simulink model "torque_reflex"  (R2019b)
settings: Solver=ode4  StartTime=0.0  StopTime=inf  FixedStep=BKIN_STEP_TIME  RelTol=1e-3  EnableMultiTasking=on
StartFcn:
  |  warndlg('Dexterit-E models cannot run under simulation. Please compile your model and run it from within Dexterit-E.');set_param(bdroot,'SimulationCommand','stop')
model workspace (MAT data in the model file):
  ACTIVE = 4
  AMPLITUDE = 7
  BASE_STIFFNESS = 12
  BKIN_KINEMATIC_FRAME_SIZE = 400
  BKIN_STEP_TIME = 0.00025
  COLOR_2 = 5
  CONDITION = 3
  DELAY_POST_TRIAL = 4
  DURATION = 5
  E_END_TRIAL = 2
  E_HAND_OUT = 4
  E_NO_EVENT = 0
  E_SHOW_TARGET = 3
  E_SRS_ON = 6
  E_START_TRIAL = 5
  E_TARGET_REACHED = 1
  HAND_OUT_TIME = 6
  IMAGE = 3
  INSERT_OFFSET = 8
  L1_LENGTH = 6
  L1_LINE = 7
  L2_LENGTH = 7
  L2_LINE = 8
  LOAD = 2
  MOVE_THRESHOLD = 10
  MUSCLE = 1
  MUSCLE_LENGTH = 1
  REFLEX = 9
  REFLEX_GAIN = 5
  RESTING_FORCE = 2
  SPEED = 6
  SPRING_X = 1
  SPRING_Y = 2
  SRS_GAIN = 13
  TARGET_1 = 3
  THICKNESS = 4
  V_MAX = 3
  WALL_DAMPING = 11
  WALL_STIFFNESS = 9
  activation = 1
  col_x = 1
  col_y = 2
undefined symbols (not defined in the file or in its folder): slselsubs
libraries: Video x5, simulink x5, xpcutilitieslib x4, KINARM_IO x4, General x3, KINARM_loads x2, KINARM_EP_loads x2, KINARM_general x1, dspstat3 x1
(part 2 of 2)

== matlab function torque_reflex/Limb Mechanics /Integrate Signals ==
  settings: fimath=|
      | fimath(...
      | 'RoundMode', 'floor',...
      | 'OverflowMode', 'wrap',...
      | 'ProductMode', 'KeepLSB', 'ProductWordLength', 32,...
      | 'SumMode', 'KeepLSB', 'SumWordLength', 32,...
      | 'CastBeforeSum', false)
  data: t_0 input; rest_length input; Force input; hand_forces output; L2_offset input; force_SRS input; d input; L2 input; spring_constant input; FS input; muscle_vector input; out_angle output; force_muscle output
function [hand_forces, out_angle, force_muscle] = hill_forces(t_0, rest_length, Force, L2_offset, force_SRS, d, L2, spring_constant, FS, muscle_vector)
% spring_force = spring_constant * (rest_length - spring_length);
% spring_force = max( min(spring_force, force_limit), -force_limit);					% limit the spring force magnitude
% F_x = spring_force * (spring_vector(1) / spring_length);		% component of force in x-direction
% F_y = spring_force * (spring_vector(2) / spring_length);		% component of force in y-direction
% F_x = Force_N * (muscle_vector(1) / muscle_length);	% component of force in x-direction
% F_y = Force_N * (muscle_vector(2)/ muscle_length); %y component
% F_x = max(min(F_x, force_limit), -force_limit);
% F_y = max(min(F_y, force_limit), -force_limit);

force_limit = 35; %Newtons

%spring_constant = load table muscle stiffness (row 11)

muscle_length = sqrt(sum(muscle_vector.^2)); %norm of the vector

muscle_diff = muscle_length - rest_length;

if muscle_diff > 0
     spring_force = spring_constant * muscle_diff; % F = k * delta_x
else
    spring_force = 0;
end
%% add up all the forces: SRS, passive (spring), active (input Force parameter)
Force = (Force * t_0) + spring_force + force_SRS; %relative tension to force in newtons, add spring force in newtons

x2 = L2_offset(1);
y2 = L2_offset(2);
x1 = 1;
y1 = 0; %horizontal line!

joint_ang = atan2(x1*y2-y1*x2,x1*x2+y1*y2); % angle between L2_vec and horizontal (??)
orth_ang = joint_ang - (pi/2); %shrink 90 degrees CCW to get angle between L1 and L2. 
orth_v = [cos(orth_ang) sin(orth_ang)]; %unit vector in direction perpindicular L2 

u = [muscle_vector, 0];
v = [L2_offset, 0]; 

theta = atan2(norm(cross(u,v)), dot(u,v));

torque_generated = Force * d * sin(theta);

Force_hand = torque_generated / L2;

%Force =Force generated by the muscle

F_x = Force_hand * orth_v(1);	% component of force in x-direction
F_y = Force_hand * orth_v(2);    %y component


out_angle = torque_generated;

force_muscle = Force; %force generated by Hill model converted to a torque at the hand ! 

FS = FS(1:2);
% proj = (dot(F_m, orth_v)/norm(orth_v)^2)*orth_v; %projection of muscle vector onto line perpindicular to L2
%(dot(A,B)/norm(B)^2)*B
C = (dot(FS,L2_offset)/norm(L2_offset)^2)*L2_offset; %vector projection of Force Sensor onto joint angle!
C = C * -1; %C is the component of Force sensor in the direction parallel to the L2 link (x,y)

F_x = F_x + C(1);
F_y = F_y + C(2); %add the reactive components to stifle lengthening/shortening of L2 length

F_x = max(min(F_x, force_limit), -force_limit);
F_y = max(min(F_y, force_limit), -force_limit);

hand_forces = [F_x, F_y, -F_x, -F_y];

== matlab function torque_reflex/Limb Mechanics /make vector  ==
  data: fla input; fla_len_out output; flp input; fv input; fla_f_out output; flp_len_out output; flp_f_out output; fv_v_out output; fv_f_out output; srs input; srs_len_out output; srs_f_out output
function [fla_len_out,fla_f_out,flp_len_out,flp_f_out,fv_v_out,fv_f_out, srs_len_out, srs_f_out] = make_vector(fla,flp, fv, srs)

persistent fla_len fla_f flp_len flp_f fv_v fv_f srs_len srs_f n;

if isempty(n)
    n = 1;
end

vector_lengths = [19, 15, 41, 20];

%     fla_len_out = [1:19]';
%     fla_f_out = zeros(19,1);
%     flp_len_out = [1:15]';
%     flp_f_out = zeros(15,1);
%     fv_v_out = [1:41]';
%     fv_f_out = zeros(41,1);

if isempty(fla_len)
    fla_len = [1:19]';
end
if isempty(fla_f)
    fla_f = zeros(19,1);
end
if isempty(flp_len)
    flp_len = [1:15]';
end
if isempty(flp_f)
    flp_f = zeros(15,1);
end
if isempty(fv_v)
    fv_v = [1:41]';
end
if isempty(fv_f)
    fv_f = zeros(41,1);
end
if isempty(srs_f)
    srs_f = zeros(20, 1);
end
if isempty(srs_len)
    srs_len = [1:20]';
end

%% overwrite vectors as data is read in!
if n <=19
    fla_len(n) = fla(1);
    fla_f(n) = fla(2);
end
if n <= 15
    flp_len(n) = flp(1);
    flp_f(n) = flp(2);
end
if n <= 41
    fv_v(n) = fv(1);
    fv_f(n) = fv(2);
end
if n <= 20
    srs_len(n) = srs(1);
    srs_f(n) = srs(2);
end

%% assign output vectors to file data once completely read!
fla_len_out = fla_len;
fla_f_out = fla_f;
flp_len_out = flp_len;
flp_f_out = flp_f;
fv_v_out = fv_v;
fv_f_out = fv_f;
srs_f_out = srs_f;
srs_len_out = srs_len;

n = n+1;

% if isempty(fla_len)
%     fla_len = [fla(1)];
% elseif length(fla_len) < 19
%     fla_len = [fla_len; fla(1)];
% end
% if isempty(fla_f)
%     fla_f = [fla(2)];
% elseif length(fla_f) < 19
%     fla_f = [fla_f; fla(2);];
% end
% if isempty(flp_len)
%     flp_len = [flp(1)];
% elseif length(flp_len) < 15
%     flp_len = [flp_len; flp(1)];
% end
% if isempty(flp_f)
%     flp_f = [flp(2)];
% elseif length(flp_f) < 15
%     flp_f = [flp_f; flp(2)];
% end
% if isempty(fv_v)
%     fv_v = [fv(1)];
% elseif length(fv_v) < 41
%     fv_v = [fv_v; fv(1)];
% end
% if isempty(fv_f)
%     fv_f = [fv(2)];
% elseif length(fv_f) < 41
%     fv_f = [fv_f; fv(2)];
% end

% if length(fla_len) == length(fla_len_out)
%     fla_len_out = fla_len;
% end
% if length(fla_f) == length(fla_f_out)
%     fla_f_out = fla_f;
% end
% if length(flp_len) == length(flp_len_out)
%     flp_len_out = flp_len;
% end
% if length(flp_f) == length(flp_f_out)
%     flp_f_out = flp_f;
% end
% if length(fv_v) == length(fv_v_out)
%     fv_v_out = fv_v;
% end
% if length(fv_f) == length(fv_f_out)
%     fv_f_out = fv_f;
% end

end

== matlab function torque_reflex/Update position of L2 shank! ==
  data: VCODE_IN input; elbow_pos input; VCODE output; handPos input
function VCODE = update_position(VCODE_IN, elbow_pos, handPos)

% This function takes a VCODE that draws a line and updates the starting and end-point of the line
% In this particular instance however, the 'line' will have a graphic pasted over it.

VCODE = VCODE_IN;

handPos1 = handPos(1, :);  %EP Hand position
handPos2 = handPos(2, :); %TWP(SPRING_X), TWP(SPRING_Y) in get_hand_pos

% update VCODE starting and endpoint positions (i.e. assumes that VCODE is for a line).
VCODE(3:4) = handPos1; %start of the line Vcode (x,y coordinates)
VCODE(10:11) = elbow_pos - handPos1;  %vector offset from start of line!
%set the relative position from one hand to the other

== matlab function torque_reflex/calibration target hold/Embedded MATLAB Function ==
  data: VCODE_IN input; SRS_state input; VCODE_OUT output; target input
function VCODE_OUT  = fcn(VCODE_IN, SRS_state, target)
%#eml
% This embedded matlab function replaces the X and Y locations of the target with constantly updated 
% positions so that the target moves in a circle in rhythm with a sine
% function

persistent moving move_counter

if isempty(moving)
    moving = 0;
end
if isempty(move_counter)
    move_counter = 0;
end

if moving == 1
    if SRS_state == 0 %this is when SRS has been inactivated i.e. a new trial. 2 means it is off for this trial. 
        moving = 0;
    end
end

if moving == 0
    if SRS_state == 1 %this is the SRS_on signal telling us the hand has been in the target for long enough. 
        moving = 1; %moving remains 1 after SRS is turned off during the trial!
    end
end

% persistent hold_counter;
% persistent hold_complete;

% if isempty(hold_complete)
%     hold_complete = 0;
% end
% 
% hold_length = hold_length * 4; %4 kHz sampling rate (!)

% if SRS_over
%     hold_complete = 0;
% end

% if isempty(hold_counter)
%     hold_counter = 0;
% else
%     if statein==2 %if hand is in the target!
%         hold_counter = hold_counter + 0.001;
%     else
%         hold_counter = 0;
%     end
% end



speed_index = 6;							% column in target table containing speed of movement
amplitude_idx = 7;							% column in target table containing radius of movement

speed = target(speed_index) * 2 * pi;		% number of radians per second
length = target(amplitude_idx) * 0.01;		% radius of circular movement (m)

VCODE_OUT = VCODE_IN; %default initialization
VCODE_OUT(3) = VCODE_IN(3); %shift X left. Y position [idx 4] is defined in TP 
VCODE_OUT(2) = 1;							% default value is that target is 'on'

if moving == 1 %target is moving
    %CODE TO MOVE IN HALF CIRCLE,
    VCODE_OUT(3) = VCODE_IN(3) + length * -abs(cos(speed * (move_counter) + (pi/2))); 	% X location of target, always negative so its only left sided
    VCODE_OUT(4) = (VCODE_IN(4) - length) + length * sin(speed * (move_counter) + (pi/2));		% Y location of target
    move_counter = move_counter + 0.00025; %
end


% HandX = hand_pos(1);
% HandY = hand_pos(2);
% deltax = HandX- VCODE_OUT(3);    % X position of target
% deltay = HandY - VCODE_OUT(4);   % Y Position of target
% 
%  radius = VCODE_OUT(10);
 %handInTarget = abs(deltax) < radius && abs(deltay) < radius;

% target_count = size(VCodes, 1);
% intarget = zeros(target_count, 1);
%% code for multiple targets (commented out)
% for n=1:target_count
%     target_type = VCodes(n, 1);
%     if target_type > 10 && target_type < 20
%         target_type = target_type - 10; %account for targets with text
%     end
%%

== matlab function torque_reflex/KINARM_HandInTarget/Embedded MATLAB InsideTarget ==
  settings: fimath=|
      | fimath(...
      | 'RoundMode', 'floor',...
      | 'OverflowMode', 'wrap',...
      | 'ProductMode', 'KeepLSB', 'ProductWordLength', 32,...
      | 'SumMode', 'KeepLSB', 'SumWordLength', 32,...
      | 'CastBeforeSum', false)
  data: handpos input size=2; VCODE_IN input; target_type input; attribcol input; num_targets input; intarget output; Target_Table input
function intarget = FIsInsideTarget(handpos, VCODE_IN, target_type, attribcol, num_targets, Target_Table)
% all dimensions in m, rad
% arguments:
% handpos: x,y positions of center of target
% attribcol: columns in target table specifying target attributes.  
% Specific to Target_Type
%	circle:
%	[X0,Y0,r...,rn] where:
%	X0,Y0 : centre of circle
%	r : logical radius of circle (i.e. radius used to determine 'in' or 'out' of target)
%	rn: logical radius of other targets (e.g. 2nd, 3rd) also specified in target row.
%   Up to 4 targets can be specified in a row
% ellipse:
%	[X0,Y0,a,b,t...,an, bn, tn] where:
%	X0,Y0 : centre of ellipse
%	a,b : major, minor radii of ellipse
%	t : rotation of ellipse in degrees
%	an,bn : major, minor radii of ellipse of other targets (e.g. 2nd, 3rd) also specified in target row
%	tn : rotation of ellipse in degrees of other targets (e.g. 2nd, 3rd) also specified in target row
%   Up to 4 targets can be specified in a row


target_col_x=1;
target_col_y=2;

x=handpos(1);
y=handpos(2);

intarget = zeros(size(Target_Table,1),5);
X0 = VCODE_IN(3);
Y0 = VCODE_IN(4);
% X0 = Target_Table(:,target_col_x)*0.01;			%Target Table sizes in cm in v1.4
% Y0 = Target_Table(:,target_col_y)*0.01;			%Target Table sizes in cm in v1.4

deltax=x-X0;
deltay=y-Y0;

if target_type==1			%circle
  
	for target=1:num_targets
		r = Target_Table(:,attribcol(target))*0.01;			%Target Table sizes in cm in v1.4
		% simple euclidean distance
		distance2 = deltax.^2 + deltay.^2;					%distance2 is the square of the distance
	    intarget(:,target) = (distance2 <= r.^2);
	end
elseif target_type==2		%ellipse
	for target=1:num_targets
	    a = Target_Table(:,attribcol(target*3-2))*0.01;			%Target Table sizes in cm in v1.4
	    b = Target_Table(:,attribcol(target*3-1))*0.01;			%Target Table sizes in cm in v1.4	
	    t = Target_Table(:,attribcol(target*3))*(pi / 180.0);	%Target Table angles in degrees in v1.4
		sint=sin(t);
		cost=cos(t);
		xrotate=deltax.*cost+deltay.*sint;		%location of x point in ellipse's coordinate frame
		yrotate=-deltax.*sint+deltay.*cost;		%location of y point in ellipse's coordinate frame
		m=yrotate./xrotate;						%slope of line between the (x,y) to (x0,y0) in ellipse's coordinate frame
		y2sq=1./(1./(m.*a).^2+1./b.^2);			%y2sq is y2^2, where y2 is the intersection of the ellipse and the (x,y) to (x0,y0) line
	    intarget(:,target) = (yrotate.^2 <= y2sq);
    end
elseif target_type==3       %rectangle
    for target=1:num_targets
        w = Target_Table(:,attribcol(target*3-2))*0.01;  %width (sizes in cm in v1.4)
        h = Target_Table(:,attribcol(target*3-1))*0.01;  %height (sizes in cm in v1.4)
        
        if attribcol(target*3) > 0
            t = Target_Table(:,attribcol(target*3))*(pi / 180.0);  %angle (angles in degrees in v1.4)
        else
            t = zeros(size(Target_Table, 1), 1);
        end

        sint=sin(t);
        cost=cos(t);

        xrotate=deltax.*cost + deltay.*sint;   %location of x point in rectangle's coordinate frame
        yrotate=-deltax.*sint + deltay.*cost;  %location of y point in rectangle's coordinate frame

        intarget(:,target) = abs(xrotate) <= w/2 & abs(yrotate) <= h/2;
    end
elseif target_type==4       %line
    for target=1:num_targets
        % treat the line like a rectangle of height h and width w
        % determine height (stroke width) in the same fashion as in Show_Target
        if attribcol(target*3-2) == 0                     %0 column index means stroke width of 0
            h = zeros(size(Target_Table, 1), 1);
        elseif attribcol(target*3-2) < 0                  %-ve column index means stroke width of 1mm
            h = ones(size(Target_Table, 1), 1) .* 0.001;
        else
            h = Target_Table(:,attribcol(target*3-2)) * 0.01;  %target table contains width in cm
        end
        
        ex = Target_Table(:,attribcol(target*3-1))*0.01;  %endpoint in x relative to start point (cm)
        ey = Target_Table(:,attribcol(target*3))*0.01;    %endpoint in y relative to start point (cm)
        
        w = sqrt(ex.^2 + ey.^2);                          %width (cm)
        
        % determine the vector from the line's midpoint to the hand position
        handx = deltax - ex/2;
        handy = deltay - ey/2;
        
        t = atan2(ey, ex);                                %calculate angle of the line (rads)
        sint = sin(t);
        cost = cos(t);
        
        xrotate = handx.*cost + handy.*sint;   %location of x point in rectangle's coordinate frame
        yrotate = -handx.*sint + handy.*cost;  %location of y point in rectangle's coordinate frame
 
        intarget(:,target) = abs(xrotate) <= w/2 & abs(yrotate) <= h/2;
    end
elseif target_type==5  % triangle
    for target=1:num_targets
        w = Target_Table(:,attribcol(target*4-3))*0.01;         %length (sizes in cm in v1.4)
        
        % If a height column of 0 is specified, make the triangle equilateral. Otherwise, use the
        % values for height and peak offset from the target table.
        if attribcol(target*4-2) > 0
            h = Target_Table(:,attribcol(target*4-2))*0.01;  %height (sizes in cm in v1.4)
            p = Target_Table(:,attribcol(target*4-1))*0.01;  %peak offset (sizes in cm in v1.4)
        else
            h = w.*sin(pi/3.0);
            p = zeros(size(Target_Table, 1), 1);
        end
        
        if attribcol(target*4) > 0
            t = Target_Table(:,attribcol(target*4))*(pi / 180.0);  %angle (angles in degrees in v1.4)
        else
            t = zeros(size(Target_Table, 1), 1);
        end
        
        sint = sin(t);
        cost = cos(t);
        
        xrotate = deltax.*cost + deltay.*sint;   %location of x point in triangle's coordinate frame
        yrotate = -deltax.*sint + deltay.*cost;  %location of y point in triangle's coordinate frame
        
        % Perform a point-in-triangle test using Barycentric coordinates.
        A = [-w/2 - p/3, -h/3];
        B = [2*p/3, 2*h/3];
        C = [w/2 - p/3, -h/3];
        
        v0 = C - A;
        v1 = B - A;
        v2 = [xrotate, yrotate] - A;

        dot00 = v0(:,1) .* v0(:,1) + v0(:,2) .* v0(:,2);
        dot01 = v0(:,1) .* v1(:,1) + v0(:,2) .* v1(:,2);
        dot02 = v0(:,1) .* v2(:,1) + v0(:,2) .* v2(:,2);
        dot11 = v1(:,1) .* v1(:,1) + v1(:,2) .* v1(:,2);
        dot12 = v1(:,1) .* v2(:,1) + v1(:,2) .* v2(:,2);

        invDenom = 1 ./ (dot00 .* dot11 - dot01 .* dot01);
        u = (dot11 .* dot02 - dot01 .* dot12) .* invDenom;
        v = (dot00 .* dot12 - dot01 .* dot02) .* invDenom;

        intarget(:,target) = (u > 0) & (v > 0) & (u + v < 1);
    end
end

== matlab function torque_reflex/Update L1 shank  ==
  data: VCODE_IN input; elbow_pos input; VCODE output; handPos input
function VCODE = update_position(VCODE_IN, elbow_pos, handPos)

% This function takes a VCODE that draws a line and updates the starting and end-point of the line
% In this particular instance however, the 'line' will have a graphic pasted over it.

VCODE = VCODE_IN;

handPos1 = handPos(1, :);  %EP Hand position
handPos2 = handPos(2, :); %TWP(SPRING_X), TWP(SPRING_Y) in get_hand_pos

% update VCODE starting and endpoint positions (i.e. assumes that VCODE is for a line).
VCODE(3:4) = elbow_pos; %start of the line Vcode (x,y coordinates)
VCODE(10:11) = handPos2 - elbow_pos;  %vector offset from start of line!
%set the relative position from one hand to the other

== matlab function torque_reflex/Limb Mechanics /Spring Force Channel L2 ==
  data: handPos input; hand_velocity input; load_tbl input; load_col input; L2 input; elbow_position input; forces output; muscle_on output
function [forces, muscle_on]  = forceChannel(handPos, hand_velocity, load_tbl, load_col, L2, elbow_position)

    persistent lastHandPosition
    if isempty(lastHandPosition),		lastHandPosition = zeros(1,2);	end
    
	forces = zeros(1, 4);
  
    hand_position = handPos(1, :);% instantaneous hand position (x,y)
    %hand2_pos = handPos(2, :); % instantaneous hand position (x, y) UNUSED
    load_row = 1;
    
    wallStiffness = load_tbl( load_row, load_col(9));
    
    wallDamping = load_tbl(load_row, load_col(11));
    c = wallDamping; 
    
    spring_vec = hand_position - elbow_position;
    spring_length = sqrt(sum(spring_vec.^2));
    
    hand1_pos_old = lastHandPosition;
    hand2_pos_old = elbow_position;
    
    spring_vector_prev = hand1_pos_old - hand2_pos_old;
    spring_length_prev = sqrt(sum(spring_vector_prev.^2)); %previous spring length

    %spring_diff = spring_length - spring_length_prev;
    spring_diff = spring_length_prev - spring_length; %this flips the sign of the velocity
    
    hand1_pos_next = hand_position(1,:);  + hand_velocity/4000;
    spring_vector_next = hand1_pos_next - elbow_position;

    timestep = 0.00025; % 1 kHz ---> 1 frame = 1/1000 seconds or 1 msec
    speed_spring = spring_diff/timestep; %instantaneous spring rate of length change in m/s. 
    unit_spring = spring_vector_next / norm(spring_vector_next); %gives unit vector along spring   
     
    x = spring_vec(1);
    y = spring_vec(2);
    
    damping_force = c * speed_spring; % SCALAR, should be positive when spring is being stretched
    damping_force_x = damping_force * unit_spring(1);
    damping_force_y = damping_force * unit_spring(2);
    spring_force = wallStiffness * (L2 - spring_length); % kx = k (l0 - L)
    
    
    displacement = L2 - spring_length;
    muscle_on = 1;
    if displacement > 0.1
        muscle_on = 0;
    end
    
        
    
	%the final forces will be spring force + viscous.
	forces(1) = spring_force * (x/spring_length) + damping_force_x;
	forces(2) = spring_force * (y / spring_length) + damping_force_y;
    forces(3) = -forces(1);
    forces(4) = -forces(2); 
    
    lastHandPosition = hand_position;
    
end

== matlab function torque_reflex/Limb Mechanics /Activation, SRS, Muscle Stiffness ==
  data: length_relative input; threshold input; SRS_on input; active input; activation output; condition input; velocity input; delay_velocity input; reflex_gain input; stretch_length output; SRS_switch output
function [activation, stretch_length, SRS_switch] = forward_control(length_relative, threshold, SRS_on, active, condition, velocity, delay_velocity, reflex_gain)

persistent rest_length start_flag
%given the condition, the velocity and the active level of activation,
%output either zero or the active activation

if isempty(rest_length)
    rest_length = 1;
end
if isempty(start_flag)
    start_flag = 0;
end

stretch_length =0 ;
activation = 0;
% moving = 0;
% SRS_on = hold_complete;

if condition == 0 %constant activation---> always on!
    activation = active;
    if abs(velocity) >= threshold
%         moving = 1;
    end
elseif condition == 1 %concentric condition, active only when velocity is negative
    if velocity <= (threshold * -1) %when velocity is negative activate muscle
        activation = active;
%         moving = 1; %track if moving so that we can turn on SRS if necessary
    else
        activation = 0;
    end
elseif condition==2 %eccentric condition, active only when velocity is positive
    if velocity >= threshold
        activation = active;
%         moving = 1;
    else
        activation = 0;
    end
elseif condition == 3 %velocity based reflex, fourth condition (!)
    
    if delay_velocity >= threshold
        reflex_act = reflex_gain * delay_velocity; %reflex activation
        reflex_act = max(reflex_act, 0); %only additive for now. 
        activation = reflex_act + active;
        stretch_length = (length_relative - rest_length)/rest_length; %???
    else
        activation = active; %Reflex is ONLY on when moving the muscle(!)
    end
end

activation = min(1, activation); %max activation = 1!

if start_flag == 0 && SRS_on %if SRS is on but we haven't switched this flag, first run through the loop
    rest_length = length_relative; %assign the resting length of the muscle
    stretch_length = 0;
    start_flag = 1;
elseif SRS_on && start_flag ==1 %we have already started SRS (start flag no longer empty/0)
    stretch_length = (length_relative - rest_length)/rest_length;
elseif (SRS_on==0) && (start_flag==1) %exited SRS !
    start_flag= 0;
    stretch_length = 0;
end
SRS_switch = 0;
if SRS_on == 2
    SRS_switch = 0;
elseif SRS_on == 0
    SRS_switch = 0;
elseif SRS_on == 1
    SRS_switch = 1;
end

== matlab function torque_reflex/Limb Mechanics /Force Channel WALL ==
  data: forces output; hand_position input; hand_velocity input; loadTable input; enable_forces input
function forces = forceChannel(hand_position, hand_velocity, loadTable, enable_forces)

	persistent lastForcesEnabledValue forceEnableTime clockCycle outsideChannel lastHandPosition;
	
	if isempty(lastForcesEnabledValue), lastForcesEnabledValue = 0;		end
	if isempty(forceEnableTime),        forceEnableTime = 1;			end
	if isempty(clockCycle),				clockCycle = 0;					end
	if isempty(outsideChannel),			outsideChannel = 0;				end
	if isempty(lastHandPosition),		lastHandPosition = zeros(1,2);	end


	%we need to keep track of the time so we can safely ramp up forces when 
	%the trial starts.
	clockCycle = clockCycle + 1;
	if lastForcesEnabledValue == 0 && enable_forces == 1
		forceEnableTime = clockCycle;
	end

	lastForcesEnabledValue = enable_forces;

	%start out assuming we will apply no forces.
	forces = zeros(1, 4);

    channelWidthM = abs((loadTable(1) * 0.01) / 2.0);%get the width of the zero force zone and convert to meters
	wallWidthM = abs(loadTable(2) * 0.01);			%get the width of the wall where forces cut out and convert to meters.
    
    % No secondary encoders
    wallStiffness = abs(loadTable(9));				%in N/m
    viscosity = -abs(loadTable(11));					%in N/(m/s)
    
	xHand=hand_position(1);		%(m)
	yHand=hand_position(2);		%(m)

	%get the target positions and convert them to meters.
% 	x1 = target1(xIdx) * 0.01;
% 	y1 = target1(yIdx) * 0.01;
% 	x2 = target2(xIdx) * 0.01;
% 	y2 = target2(yIdx) * 0.01;
    
    x1 = 0;
    y1 = 0.52;
    x2 = 0;
    y2 = 0;
    

	%http://www.codeguru.com/forum/showthread.php?threadid=194400
	%This calculations gives us the distance away from the line we are now.
	distToLine = abs(((x2 - x1)*(y1-yHand)) - ((x1 - xHand)*(y2-y1))) / sqrt( (x2 - x1)^2 + (y2 - y1)^2 );

	HXVEL = hand_velocity(1);
	HYVEL = hand_velocity(2);
	viscosityX = HXVEL * viscosity;
	viscosityY = HYVEL * viscosity;

	%we only ever want to provide a viscous load perpendicular to
	%the force channel. This viscous force will be used to dampen
	%any instability.
	if (x2 == x1) %infinite slope
		viscosityY = 0;	
	elseif (y2 == y1) %0 slope
		viscosityX = 0;
	else
		m = (y2 - y1) / (x2 - x1);
		perpM = -(1/m);	

		%we need to scale the viscous load to only the components
		%that are perpendicular to the line. To do that we find the 
		%projection of the velocity vecotor on a line perpendicular to the
		%force channel
		perpVect = [1 perpM];
		perpUnitVector = perpVect / norm(perpVect);

		%this finds the projection of the vector perpendicular to the channel
		dotProduct = dot([viscosityX viscosityY], perpUnitVector);
		scaledForces = dotProduct * perpUnitVector;

		viscosityX = scaledForces(1);
		viscosityY = scaledForces(2);
	end

	%forces 1,2 are for right arm, 3,4 are for left
	% if we are outside the force wall we need to make sure we don't turn it
	%back on until we are in the channel. Otherwise it's quite jarring to be pulled in.
	if distToLine > (wallWidthM + channelWidthM)
		outsideChannel = 1;
		return
	elseif enable_forces == 0
		return	
	%if we are in the force channel we still need to viscous loads to aid in stability
	%if we are bouncing between the walls. 
	elseif distToLine < channelWidthM 
		outsideChannel = 0; %we're in the channel, so we can turn forces back on if they were off.
		return
	elseif outsideChannel == 1    
		%If we were outside the wall then forces are all off. We only want to turn
		%forces back on if the hand has crossed the line of the force channel, that way
		%you are not pushed into the channel, it only feels like you hit a wall.
		%By looking at the previous hand position and the current hand position
		%we can see if that line segment crosses the channel line, in which case we can
		%turn the forces back on.
		if doLinesIntersect([x1 y1], [x2 y2], [xHand yHand], lastHandPosition) == 1
			outsideChannel = 0;
		else
			return
		end
	end

	distIntoWall = distToLine - channelWidthM;

	if (x2 == x1) %all force wille be in x direction
		y = 0;
		if xHand < x1
			x = distIntoWall;
		else
			x = -distIntoWall;
		end
	elseif (y2 == y1) %all force will be in Y direction
		x = 0;
		if yHand < y1
			y = distIntoWall;
		else
			y = -distIntoWall;
		end	
	else
		%we need to find out how far off the line in X and Y we are in meters so 
		%we can properly convert the wall stiffness in N/m to a force.
		m = (y2 - y1) / (x2 - x1);
		b = y1 - (m * x1);

		perpM = -(1/m);	
		perpB = yHand - (perpM * xHand);

		xIntersect = (b - perpB) / (perpM - m);
		yIntersect = (m * xIntersect) + b;

		%x and y are converted to distances in meters from the center line
		x = xIntersect - xHand;
		y = yIntersect - yHand;

		%take the distances from center and convert to a unit vector,
		%then multiply by the distance to where the forces start
		%this gives us a clean number to use when calculating wall force.
		x = (x / sqrt(x^2 + y^2)) * distIntoWall;
		y = (y / sqrt(x^2 + y^2)) * distIntoWall;
	end

	%we don't want to just shut off the forces, we need to ramp them down
	%somewhat. This finds out how far into the wall we are and allows us
	%to ramp down the forces over the last 25% of the wll.
	forceRampDownZoneSizePercent = 0.75; %start ramping down the forces in the last 25% of the wall
	forceMaxEndLocInWallM = forceRampDownZoneSizePercent * wallWidthM;
	distanceIntoWall = distToLine - channelWidthM;
	scaleWallForce = 1; %assume we can run at full calculated wall force

	if distanceIntoWall > forceMaxEndLocInWallM   %we are in the ramp down zone
		distIntoRampDownZone = distanceIntoWall - forceMaxEndLocInWallM;
		rampDownZoneWidth = wallWidthM  - forceMaxEndLocInWallM;
		scaleWallForce = (rampDownZoneWidth - distIntoRampDownZone) / rampDownZoneWidth;
	end

	%within the first 1.5 seconds of the trial we don't want to jar anyone
	%this ramps the forces up slowly so you get a gentle nudge into
	%the force channel, not a violent jerk.
	timeDelta = clockCycle - forceEnableTime;
	timeScaling = 1;
	if (timeDelta < 1500)
		timeScaling = timeDelta / 1500.0;
	end

	%the final forces will be wall force + viscous.
	forces(1) = (wallStiffness * scaleWallForce * timeScaling * x) + viscosityX;
	forces(2) = (wallStiffness * scaleWallForce  * timeScaling * y) + viscosityY;

	lastHandPosition(1) = xHand;
	lastHandPosition(2) = yHand;
end

function bIntersect = doLinesIntersect(Ap1, Ap2, Bp1, Bp2)
    %This method for finding out if 2 lines segements intersect comes from:
    %http://stackoverflow.com/questions/563198/how-do-you-detect-where-two-line-segments-intersect
   	e = Ap2-Ap1;
    f = Bp2-Bp1;
    p = [-e(2) e(1)];
    h = dot((Ap1 - Bp1), p) / dot (f, p);
    
    if h >=0 && h <= 1
        bIntersect = 1;
    else
        bIntersect = 0;
    end
end

== matlab function torque_reflex/Limb Mechanics /Constant Loads ==
  settings: fimath=|
      | fimath(...
      | 'RoundMode', 'floor',...
      | 'OverflowMode', 'wrap',...
      | 'ProductMode', 'KeepLSB', 'ProductWordLength', 32,...
      | 'SumMode', 'KeepLSB', 'SumWordLength', 32,...
      | 'CastBeforeSum', false)
  data: handPos input; load_tbl input; load_col input; hand_forces output; load_row input
function hand_forces  = const_loads(handPos, load_tbl, load_col, load_row)
%
% MULTI-PURPOSE SPRING between 2 hands
%
% Cleaned up for demo purposes, May 2013.

%The resting length, spring constant and force limit are passed in via the load table.
rest_length = 0;				% default rest length (m)
spring_constant = 0;			% default spring constant (N/m)
force_limit = 20;				% default force limit (N)


hand1_pos = handPos(1, :);
hand2_pos = handPos(2, :);

spring_vector = hand1_pos - hand2_pos;
spring_length = sqrt( sum( spring_vector.^2 ) );
% The first entry specifed in the load table is the resting length of the spring(m)
% The second value is the spring constant with units of N/m

if load_row > 0 && load_row <= size(load_tbl,1)
    if load_col(1) > 0
        rest_length = abs(load_tbl( load_row, load_col(1)));
    end
    if load_col(2) > 0
        spring_constant = load_tbl( load_row, load_col(2));
        %Safety limit to keep the KINARM from going unstable
        if spring_constant > 500
            spring_constant = 500;
        end
    end
    if load_col(3) > 0
        force_limit = load_tbl( load_row, load_col(3));
		force_limit = abs(force_limit);						%force the limit to positive
	end
end

% Positive force indicates the spring is in compression so the arms will be pushed outwards
spring_force = spring_constant * (rest_length - spring_length);
spring_force = max( min(spring_force, force_limit), -force_limit);					% limit the spring force magnitude
F_x = spring_force * (spring_vector(1) / spring_length);		% component of force in x-direction
F_y = spring_force * (spring_vector(2) / spring_length);		% component of force in y-direction

hand_forces = [F_x, F_y, -F_x, -F_y] ;
